simulink model "ofdmdemo2"  (Simulink 10.1)
settings: Solver=ode45  StartTime=0.0  StopTime=10000.0  RelTol=1e-3  EnableMultiTasking=on
libraries: dspxfrm3 x2, simulink x2, commdigbbndpm3 x2, commsink2 x1
settings Model: Creator=tmiyagi  LastModifiedBy=tsudashouki  ExtModeTrigMode=oneshot  ExtModeArmWhenConnect=off
settings DataIOCC: SignalLoggingSaveFormat=ModelDataLogs
settings OptimizationCC: BlockReduction=off  BooleanDataType=off  ExpressionDepthLimit=2147483647
settings DebuggingCC: SaveWithParameterizedLinksMsg=none  SignalResolutionControl=TryResolveAllWithWarning  MultiTaskDSMMsg=warning  MultiTaskCondExecSysMsg=none  FcnCallInpInsideContextMsg=warning  StateNameClashWarn=warning
settings HardwareCC: TargetUnknown=on

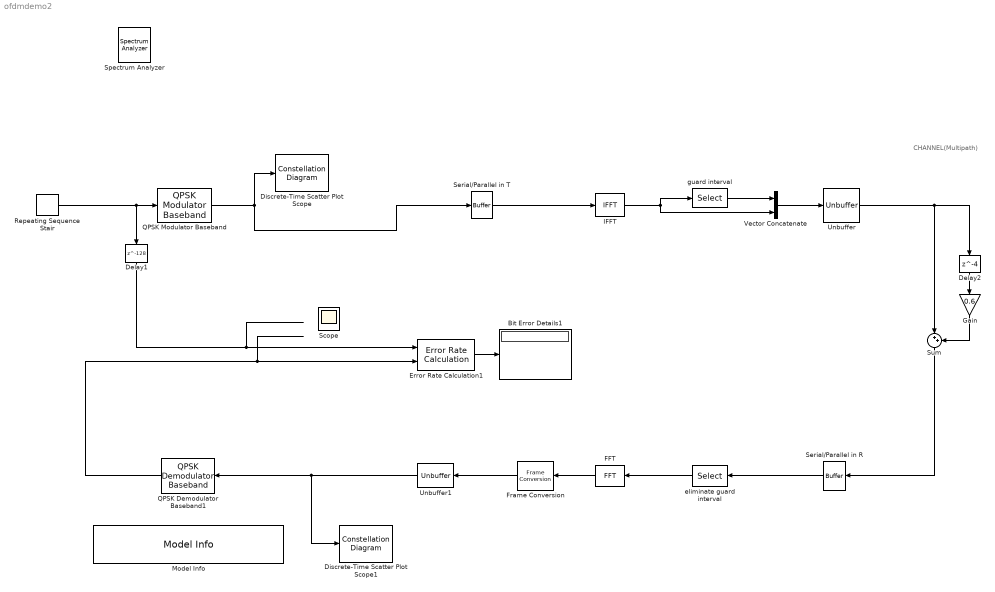
== system ofdmdemo2 ==
  note: CHANNEL(Multipath)
  " Delay1" : Delay  DelayLength=128
  " Delay2" : Delay  DelayLength=4  InitialCondition=0
  Bit Error Details1 : Display
  Discrete-Time Scatter Plot Scope : ConstellationDiagram  Tag=ScatterPlot
  Discrete-Time Scatter Plot Scope1 : ConstellationDiagram  Tag=ScatterPlot
  Error Rate Calculation1 : commsink2/Error Rate Calculation  N=0  st_delay=0  cp_mode=Entire frame  subframe=[]  PMode=Port  WsName=ErrorVec  RsMode2=off  stop=off  numErr=100  maxBits=1e6
  FFT : dspxfrm3/FFT  FFTImplementation=Auto  CompMethod=Table lookup  TableOpt=NEW  TableOptActive=Speed  BitRevOrder=off  Normalize=off  InheritFFTLength=on  FFTLength=64  WrapInput=on  roundingMode=Floor  overflowMode=off  firstCoeffDataTypeStr=Inherit: Same word length as input  firstCoeffLastDataTypeStr=Inherit: Same word length as input  outputMin=[]  outputMax=[]
  Frame Conversion : FrameConversion
  Gain : Gain  Gain=0.6  SaturateOnIntegerOverflow=on  OutDataTypeStr=Inherit: Same as input  ParamDataTypeStr=Inherit: Same as input
  IFFT : dspxfrm3/IFFT  FFTImplementation=Auto  CompMethod=Table lookup  TableOpt=NEW  TableOptActive=Speed  BitRevOrder=off  cs_in=off  Normalize=on  InheritFFTLength=on  FFTLength=64  WrapInput=on  mode=Complex  outSamplingMode=Frame based  roundingMode=Floor  overflowMode=off  firstCoeffDataTypeStr=Inherit: Same word length as input  firstCoeffLastDataTypeStr=Inherit: Same word length as input  outputMin=[]  outputMax=[]
  Model Info : simulink/Model-Wide Utilities/Model Info  Frame=off  DisplayStringWithTags=|  HorizontalTextAlignment=Left  LeftAlignmentValue=0.02
      | %<ModifiedDate> 16-OFDM system and Equlizer
      | %<Creator> Tomohide Miyagi
      | Add guard interval signal
      | Proposed Equalizer
  QPSK Demodulator Baseband1 : commdigbbndpm3/QPSK Demodulator Baseband  OutType=Integer  DecType=Hard decision  VarSource=Dialog  Variance=1  Dec=Gray  Ph=pi/4  outDtype1=Inherit via internal rule  outDtype2=Inherit via internal rule  derotateFactorWordLen=16  derotateFactorDataTypeStr=Inherit: Same word length as input  derotateFactorLastDataTypeStr=Inherit: Same word length as input
  QPSK Modulator Baseband : commdigbbndpm3/QPSK Modulator Baseband  InType=Integer  Enc=Gray  Ph=pi/4  outDtype=double  outWordLen=16  outUDDataType=sfix(16)  outFracLenMode=Best precision  outFracLen=15  outDataTypeStr=double  outLastDataTypeStr=double
  Repeating Sequence Stair : simulink/Sources/Repeating Sequence Stair  OutValues=randi(4,1000,1) -1  tsamp=1  OutMin=[]  OutMax=[]  OutDataTypeStr=Inherit: Inherit via back propagation  OutDataType=double  ConRadixGroup=Best Precision: Vector-wise  OutScaling=2^-12
  Scope : Scope
  Serial/Parallel in R : Buffer  N=64+16
  Serial/Parallel in T : Buffer
  Sum : Sum  Inputs=|++  InputSameDT=on  SaturateOnIntegerOverflow=on  OutDataTypeStr=Inherit: Same as first input
  Unbuffer : Unbuffer
  Unbuffer1 : Unbuffer
  Vector Concatenate : Concatenate  Mode=Multidimensional array
  eliminate guard interval : Selector  InputPortWidth=64+16  IndexOptions=Index vector (dialog)  Indices=[17:64+16]  OutputSizes=1
  guard interval : Selector  InputPortWidth=64  IndexOptions=Index vector (dialog)  Indices=[49:64]  OutputSizes=1
  Spectrum Analyzer : SpectrumAnalyzer  IOType=viewer
  wires:
  QPSK Modulator Baseband/1 -> Discrete-Time Scatter Plot Scope/1, Serial/Parallel in T/1
  Repeating Sequence Stair/1 -> QPSK Modulator Baseband/1, " Delay1"/1
  Serial/Parallel in T/1 -> IFFT/1
  IFFT/1 -> guard interval/1, Vector Concatenate/2
  guard interval/1 -> Vector Concatenate/1
  Unbuffer/1 -> Sum/1, " Delay2"/1
  Sum/1 -> Serial/Parallel in R/1
  Vector Concatenate/1 -> Unbuffer/1
  Serial/Parallel in R/1 -> eliminate guard interval/1
  eliminate guard interval/1 -> FFT/1
  FFT/1 -> Frame Conversion/1
  Error Rate Calculation1/1 -> Bit Error Details1/1
  QPSK Demodulator Baseband1/1 -> Error Rate Calculation1/2
  Frame Conversion/1 -> Unbuffer1/1
  Unbuffer1/1 -> QPSK Demodulator Baseband1/1, Discrete-Time Scatter Plot Scope1/1
  " Delay2"/1 -> Gain/1
  Gain/1 -> Sum/2
  " Delay1"/1 -> Error Rate Calculation1/1
